simulink model "Rectifiers"  (R2023b)
settings: Solver=VariableStepAuto  StartTime=0.0  StopTime=0.1  RelTol=1e-3
values from neighbouring files (symbols this model uses):
  sys = Sources()    [Main.m]
libraries: spsVoltageMeasurementLib x8, spsDiodeLib x5, spsACVoltageSourceLib x4, spsCurrentMeasurementLib x4, spsSeriesRLCBranchLib x4, spsThyristorLib x4, spsDetailedThyristorLib x1, sps_lib x1
settings Model: Creator=JesperBertelsen  LastModifiedBy=JesperBertelsen

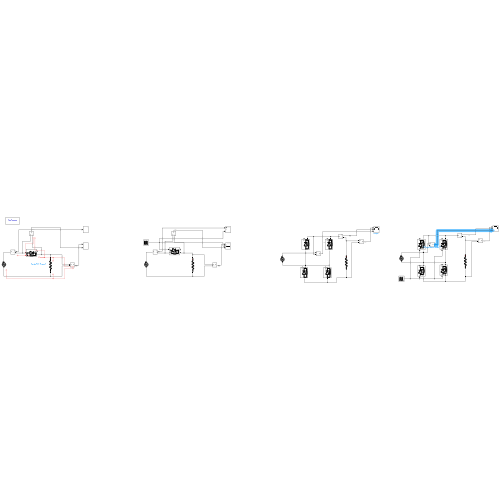
[thumbnail: Simulink's stored preview of the top-level diagram]
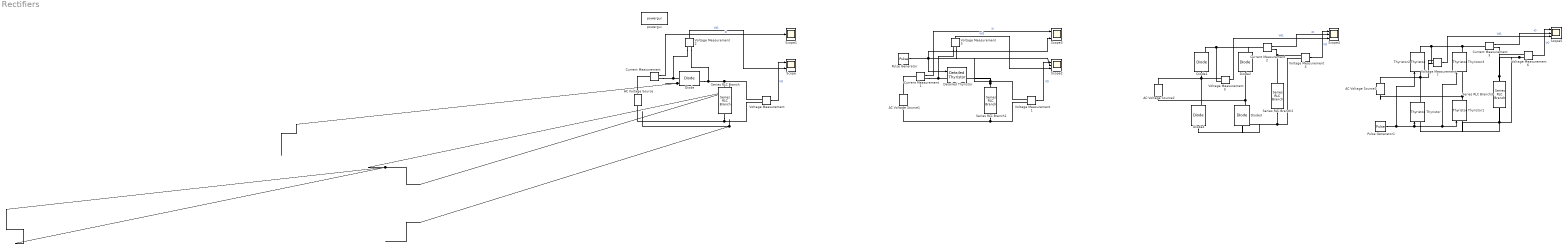
== system Rectifiers ==
  AC Voltage Source{,1..3} (4 alike) : spsACVoltageSourceLib/AC Voltage Source  Amplitude=400*sys.Vm*sqrt(2)  Phase=0  Frequency=60  SampleTime=0  Measurements=None  BusType=swing  Pref=10e3  Qref=0  Qmin=-inf  Qmax=+inf
  Current Measurement{,1..3} (4 alike) : spsCurrentMeasurementLib/Current Measurement  PhasorSimulation=off  OutputType=Complex  PSBequivalent=0
  Detailed Thyristor : spsDetailedThyristorLib/Detailed Thyristor  Ron=0.001  Lon=1e-3  Vf=0.8  IL=0.1  Tq=100e-6  IC=0  Rs=500  Cs=250e-9  Measurements=on
      settings: LibrarySourceBlock=sps_lib/Power Electronics/Detailed Thyristor
  Diode{,1..4} (5 alike) : spsDiodeLib/Diode  Ron=0.001  Lon=0  Vf=0.8  IC=0  UseSnubber=0  Rs=500  Cs=250e-9  Measurements=on
  Pulse Generator : DiscretePulseGenerator  PulseType=Time based  Period=1/60  PulseWidth=60/360
  Pulse Generator1 : DiscretePulseGenerator  PulseType=Time based  Period=1/60  PulseWidth=60/360
  Scope : Scope  NumInputPorts=2
  Scope1 : Scope
  Scope2 : Scope  NumInputPorts=3
  Scope3 : Scope  NumInputPorts=2
  Scope4 : Scope  NumInputPorts=3
  Scope5 : Scope  NumInputPorts=3
  Series RLC Branch{,1..3} (4 alike) : spsSeriesRLCBranchLib/Series RLC Branch  LConnTagsString=__new0  RConnTagsString=__new0  BranchType=R  Resistance=sys.R  Inductance=1e-3  SetiL0=off  InitialCurrent=0  Capacitance=1e-6  Setx0=off  InitialVoltage=0  Measurements=None
  Thyristor{,1..3} (4 alike) : spsThyristorLib/Thyristor  Ron=0.001  Lon=0  Vf=0.8  IC=0  Rs=500  Cs=250e-9  Measurements=on
  Voltage Measurement{,1..7} (8 alike) : spsVoltageMeasurementLib/Voltage Measurement  PhasorSimulation=off  OutputType=Complex  PSBequivalent=0
  powergui : sps_lib/powergui  Priority=1  SimulationMode=Continuous  SampleTime=50e-6  frequency=60  Iterations=50  frequencyindice=60  Pbase=100e6  ErrMax=1e-4  UnitsV=kV  UnitsW=MW  buscounter=0  FunctionMessages=off  echomessages=off  EnableUseOfTLC=off  CurrentSourceSwitches=off  DisableSnubberDevices=off  DisableRonSwitches=off  DisableVfSwitches=off  DisplayEquations=off  AutomaticDiscreteSolvers=off  SolverType=Tustin/Backward Euler (TBE)  Interpol=off  ExternalGateDelay=off  methode=off  Ts=100  x0status=blocks  SPID=on  SwTol=0  HookPort=off  NonlinearTolerance=1e-4  nMaxIteration=100  ContinueOnMaxIteration=off  RestoreLinks=warning  ResistiveCurrentMeasurement=off  Frange=[0:2:500]  Ylog=off  Xlog=on  ShowGrid=off  save=off  variable=ZData  structure=0  ZoomFFT=off  StartTime=0.0  cycles=1  DisplayStyle=1  fundamental=60  FreqAxis=off  MaxFrequency=1000  frequencyindicesteady=1  RmsSteady=1  display=off
  wires:
  Voltage Measurement/1 -> Scope/1  "VO"
  Voltage Measurement2/1 -> Scope/2  "Vd1"
  Current Measurement/1 -> Scope1/1  "i0"
  Voltage Measurement1/1 -> Scope2/1  "VO"
  Current Measurement1/1 -> Scope3/1  "i0"
  Voltage Measurement3/1 -> Scope2/3  "Vd1"
  Pulse Generator/1 -> Detailed Thyristor/1, Scope2/2, Scope3/2
  Voltage Measurement4/1 -> Scope4/1  "VO"
  Voltage Measurement5/1 -> Scope4/3  "Vd1"
  Current Measurement2/1 -> Scope4/2  "iO"
  Voltage Measurement6/1 -> Scope5/1  "VO"
  Current Measurement3/1 -> Scope5/2  "iO"
  Pulse Generator1/1 -> Thyristor2/1, Thyristor3/1, Thyristor1/1, Thyristor/1
  Voltage Measurement7/1 -> Scope5/3  "Vd1"
  connections:
  AC Voltage Source/RConn1 -- Current Measurement/LConn1
  Series RLC Branch/RConn1 -- Voltage Measurement/LConn2 -- AC Voltage Source/LConn1
  Current Measurement/RConn1 -- Voltage Measurement2/LConn1 -- Diode/LConn1
  Diode/RConn1 -- Voltage Measurement2/LConn2 -- Voltage Measurement/LConn1 -- Series RLC Branch/LConn1
  Current Measurement1/RConn1 -- Detailed Thyristor/LConn1 -- Voltage Measurement3/LConn1
  Series RLC Branch1/LConn1 -- Voltage Measurement3/LConn2 -- Detailed Thyristor/RConn1 -- Voltage Measurement1/LConn1
  Series RLC Branch1/RConn1 -- Voltage Measurement1/LConn2 -- AC Voltage Source1/LConn1
  Current Measurement1/LConn1 -- AC Voltage Source1/RConn1
  Diode1/RConn1 -- Voltage Measurement5/LConn2 -- Current Measurement2/LConn1 -- Diode2/RConn1
  Diode1/LConn1 -- AC Voltage Source2/RConn1 -- Voltage Measurement5/LConn1 -- Diode4/RConn1
  Series RLC Branch2/RConn1 -- Diode4/LConn1 -- Diode3/LConn1 -- Voltage Measurement4/LConn2
  Diode3/RConn1 -- Diode2/LConn1 -- AC Voltage Source2/LConn1
  Voltage Measurement4/LConn1 -- Current Measurement2/RConn1 -- Series RLC Branch2/LConn1
  ?
  ?
  ?
  Series RLC Branch3/LConn1 -- Voltage Measurement6/LConn1 -- Current Measurement3/RConn1
  Voltage Measurement6/LConn2 -- Thyristor1/LConn1 -- Thyristor/LConn1 -- Series RLC Branch3/RConn1
  Thyristor1/RConn1 -- AC Voltage Source3/LConn1 -- Thyristor3/LConn1
  Thyristor/RConn1 -- Voltage Measurement7/LConn1 -- AC Voltage Source3/RConn1 -- Thyristor2/LConn1
  Thyristor2/RConn1 -- Voltage Measurement7/LConn2 -- Thyristor3/RConn1 -- Current Measurement3/LConn1
